simulink model "busrelay"  (Simulink 8.5)
settings: Solver=ode15s  SolverMode=SingleTasking  StartTime=0.0  StopTime=0.08  RelTol=1e-3  AbsTol=1e-6
libraries: powerlib_extras x27, elements x12
settings Model: Creator=PC  LastModifiedBy=PC  ExtModeTrigMode=oneshot  ExtModeArmWhenConnect=off
settings DataIOCC: LimitDataPoints=off
settings OptimizationCC: BlockReduction=off  BooleanDataType=off  ExpressionDepthLimit=128
settings DebuggingCC: SaveWithParameterizedLinksMsg=none  SignalResolutionControl=TryResolveAllWithWarning  MultiTaskDSMMsg=warning  MultiTaskCondExecSysMsg=none  FcnCallInpInsideContextMsg=EnableAllAsError  StateNameClashWarn=none  StrictBusMsg=None
settings HardwareCC: TargetUnknown=on

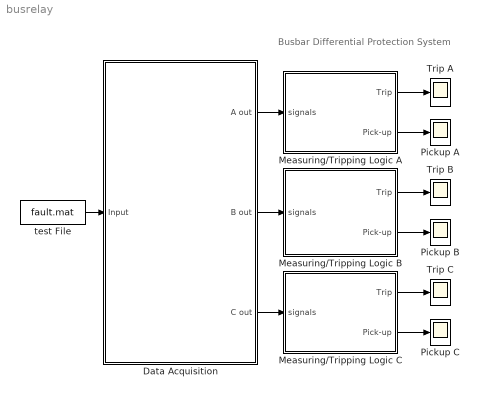
== system busrelay ==
  note: Busbar Differential Protection System
  Data Acquisition : Subsystem  mask(Data Acquisition Board){FreqSampling=60*20, FreqCutoff=360}
      mask prompts: FreqSampling "Sampling Frequecny (Hz) :"; FreqCutoff "Cut-off Frequency (Hz) :"
      mask Display: disp(' Data\nAcquistion\nBlock')
  Measuring/Tripping Logic A : Subsystem  mask(Biased Differential Relay){A0=0.2, Inorm=1, K=0.3, C1=0.1}
      mask prompts: A0 "Pickup Setting, A0 (pu):"; Inorm "Normal Load Current, Inorm (A) :"; K "Bias Setting, K (pu) :"; C1 "Harmonic Restrain Settging, C1 (pu)"
      mask help: coming soon ...
  Measuring/Tripping Logic B : Subsystem  mask(Biased Differential Relay){A0=0.2, Inorm=1, K=0.3, C1=0.1}
      mask prompts: A0 "Pickup Setting, A0 (pu):"; Inorm "Normal Load Current, Inorm (A) :"; K "Bias Setting, K (pu) :"; C1 "Harmonic Restrain Settging, C1 (pu)"
      mask help: coming soon ...
  Measuring/Tripping Logic C : Subsystem  mask(Biased Differential Relay){A0=0.2, Inorm=1, K=0.3, C1=0.1}
      mask prompts: A0 "Pickup Setting, A0 (pu):"; Inorm "Normal Load Current, Inorm (A) :"; K "Bias Setting, K (pu) :"; C1 "Harmonic Restrain Settging, C1 (pu)"
      mask help: coming soon ...
  Pickup A : Scope
      settings: TickLabels=on  YMin=0  YMax=2
  Pickup B : Scope
      settings: TickLabels=on  YMin=0  YMax=2
  Pickup C : Scope
      settings: TickLabels=on  YMin=0  YMax=2
  Trip A : Scope
      settings: TickLabels=on  YMin=0  YMax=2
  Trip B : Scope
      settings: TickLabels=on  YMin=0  YMax=1
  Trip C : Scope
      settings: TickLabels=on  YMin=0  YMax=1
  test File : FromFile  FileName=fault.mat  SampleTime=0
  wires:
  Measuring/Tripping Logic A/1(Trip) -> Trip A/1
  Measuring/Tripping Logic A/2(Pick-up) -> Pickup A/1
  test File/1 -> Data Acquisition/1("Input ")
  Data Acquisition/1(A out) -> Measuring/Tripping Logic A/1(signals)
  Measuring/Tripping Logic B/1(Trip) -> Trip B/1
  Measuring/Tripping Logic B/2(Pick-up) -> Pickup B/1
  Measuring/Tripping Logic C/1(Trip) -> Trip C/1
  Measuring/Tripping Logic C/2(Pick-up) -> Pickup C/1
  Data Acquisition/2(" B out") -> Measuring/Tripping Logic B/1(signals)
  Data Acquisition/3(C out) -> Measuring/Tripping Logic C/1(signals)

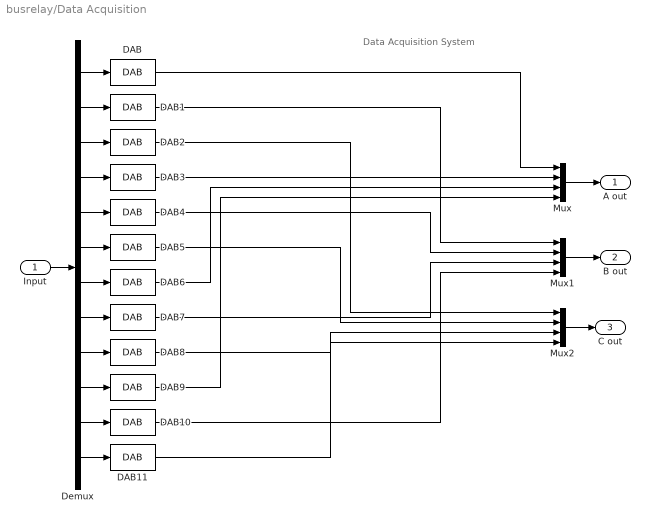
== system busrelay/Data Acquisition ==
  note: Data Acquisition System
  "Input " : Inport
  DAB{,1..11} (12 alike) : elements/DAB  filter=off  approx=Bessel  order=2  numerator=[]  denominator=[]  freq=FreqCutoff  resdis=off  vertres=12  xmax=10  winsize=1  G=1.0  fs=FreqSampling
  Demux : Demux  Outputs=12
  Mux : Mux
  Mux1 : Mux
  Mux2 : Mux
  A out : Outport
  " B out" : Outport  Port=2
  C out : Outport  Port=3
  wires:
  "Input "/1 -> Demux/1
  Mux/1 -> A out/1
  Mux2/1 -> C out/1
  Mux1/1 -> " B out"/1
  Demux/1 -> DAB/1
  DAB/1 -> Mux/1
  Demux/2 -> DAB1/1
  DAB1/1 -> Mux1/1
  Demux/3 -> DAB2/1
  DAB2/1 -> Mux2/1
  Demux/4 -> DAB3/1
  DAB3/1 -> Mux/2
  Demux/5 -> DAB4/1
  DAB4/1 -> Mux1/2
  Demux/6 -> DAB5/1
  DAB5/1 -> Mux2/2
  Demux/7 -> DAB6/1
  DAB6/1 -> Mux/3
  Demux/8 -> DAB7/1
  DAB7/1 -> Mux1/3
  Demux/9 -> DAB8/1
  Demux/10 -> DAB9/1
  DAB9/1 -> Mux/4
  Demux/11 -> DAB10/1
  DAB10/1 -> Mux1/4
  Demux/12 -> DAB11/1
  DAB11/1 -> Mux2/4
  DAB8/1 -> Mux2/3

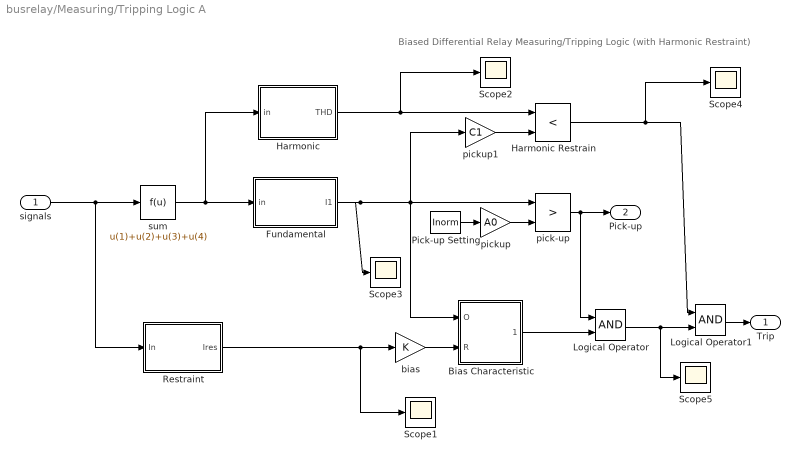
== system busrelay/Measuring/Tripping Logic A ==
  note: Biased Differential Relay Measuring/Tripping Logic (with Harmonic Restraint)
  signals : Inport
  Bias Characteristic : Subsystem  mask(Bias Characteristic){BC=[0 0;0 0.3; 0.1 0.8 ;7 4.2], fs=60*20}
      mask prompts: BC "Bias characteristic"; fs "Sampling frequency [samples per cycle]"
      mask help: Compares its two input signals using a bias characteristic. This characteristic is defined point-by-point.
      mask init:
      | bc2
      mask Display:
      | plot([xo xo],[yo y1]);
      | plot([xo x1],[yo yo]);
      | 
      | 
      | plot(R,O);
  Fundamental : Subsystem
  Harmonic : Subsystem
  Harmonic Restrain : RelationalOperator  Operator=<  InputSameDT=on
  Logical Operator : Logic
  Logical Operator1 : Logic
  Pick-up Setting : Constant  Value=Inorm
  Restraint : Subsystem
  Scope{1..5} (5 alike) : Scope
      settings: TickLabels=on  YMin=0  YMax=1
  bias : Gain  Gain=K  SaturateOnIntegerOverflow=on  OutDataTypeStr=Inherit: Same as input  ParamDataTypeStr=Inherit: Same as input
  pick-up : RelationalOperator  Operator=>  InputSameDT=on
  pickup : Gain  Gain=A0  SaturateOnIntegerOverflow=on  OutDataTypeStr=Inherit: Same as input  ParamDataTypeStr=Inherit: Same as input
  pickup1 : Gain  Gain=C1  SaturateOnIntegerOverflow=on  OutDataTypeStr=Inherit: Same as input  ParamDataTypeStr=Inherit: Same as input
  sum : Fcn  Expr=u(1)+u(2)+u(3)+u(4)
  Trip : Outport
  Pick-up : Outport  Port=2
  wires:
  signals/1 -> sum/1, Restraint/1(In)
  bias/1 -> Bias Characteristic/2(R)
  Restraint/1(Ires) -> bias/1, Scope1/1
  Bias Characteristic/1(" ") -> Logical Operator/2
  sum/1 -> Harmonic/1(in), Fundamental/1(in)
  pickup1/1 -> Harmonic Restrain/2
  Logical Operator1/1 -> Trip/1
  Pick-up Setting/1 -> pickup/1
  pickup/1 -> pick-up/2
  pick-up/1 -> Pick-up/1, Logical Operator/1
  Harmonic/1(THD) -> Harmonic Restrain/1, Scope2/1
  Fundamental/1(I1) -> pick-up/1, Bias Characteristic/1(O), pickup1/1, Scope3/1
  Harmonic Restrain/1 -> Logical Operator1/1, Scope4/1
  Logical Operator/1 -> Logical Operator1/2, Scope5/1

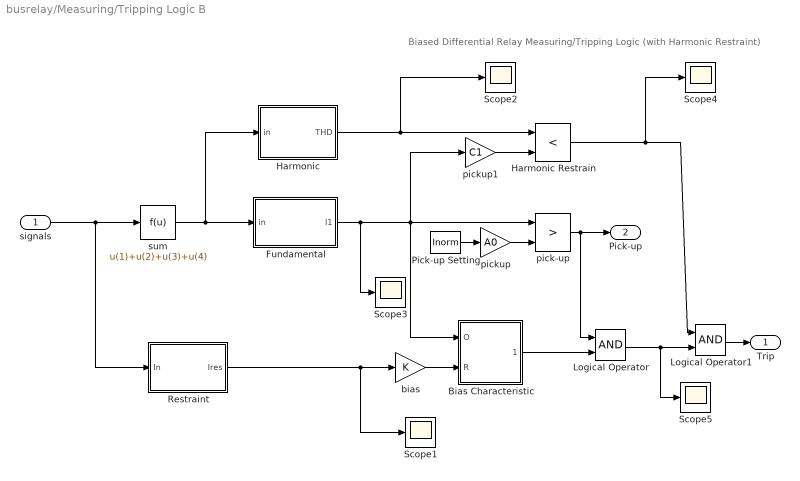
== system busrelay/Measuring/Tripping Logic B ==
  note: Biased Differential Relay Measuring/Tripping Logic (with Harmonic Restraint)
  signals : Inport
  Bias Characteristic : Subsystem  mask(Bias Characteristic){BC=[0 0;0 0.3; 0.1 0.8 ;7 4.2], fs=60*20}
      mask prompts: BC "Bias characteristic"; fs "Sampling frequency [samples per cycle]"
      mask help: Compares its two input signals using a bias characteristic. This characteristic is defined point-by-point.
      mask init:
      | bc2
      mask Display:
      | plot([xo xo],[yo y1]);
      | plot([xo x1],[yo yo]);
      | 
      | 
      | plot(R,O);
  Fundamental : Subsystem
  Harmonic : Subsystem
  Harmonic Restrain : RelationalOperator  Operator=<  InputSameDT=on
  Logical Operator : Logic
  Logical Operator1 : Logic
  Pick-up Setting : Constant  Value=Inorm
  Restraint : Subsystem
  Scope{1..5} (5 alike) : Scope
      settings: TickLabels=on  YMin=0  YMax=1
  bias : Gain  Gain=K  SaturateOnIntegerOverflow=on  OutDataTypeStr=Inherit: Same as input  ParamDataTypeStr=Inherit: Same as input
  pick-up : RelationalOperator  Operator=>  InputSameDT=on
  pickup : Gain  Gain=A0  SaturateOnIntegerOverflow=on  OutDataTypeStr=Inherit: Same as input  ParamDataTypeStr=Inherit: Same as input
  pickup1 : Gain  Gain=C1  SaturateOnIntegerOverflow=on  OutDataTypeStr=Inherit: Same as input  ParamDataTypeStr=Inherit: Same as input
  sum : Fcn  Expr=u(1)+u(2)+u(3)+u(4)
  Trip : Outport
  Pick-up : Outport  Port=2
  wires:
  Logical Operator/1 -> Scope5/1, Logical Operator1/2
  Harmonic Restrain/1 -> Scope4/1, Logical Operator1/1
  Fundamental/1(I1) -> Scope3/1, pickup1/1, Bias Characteristic/1(O), pick-up/1
  Harmonic/1(THD) -> Scope2/1, Harmonic Restrain/1
  pick-up/1 -> Logical Operator/1, Pick-up/1
  pickup/1 -> pick-up/2
  Pick-up Setting/1 -> pickup/1
  Logical Operator1/1 -> Trip/1
  pickup1/1 -> Harmonic Restrain/2
  sum/1 -> Fundamental/1(in), Harmonic/1(in)
  Bias Characteristic/1(" ") -> Logical Operator/2
  Restraint/1(Ires) -> Scope1/1, bias/1
  bias/1 -> Bias Characteristic/2(R)
  signals/1 -> Restraint/1(In), sum/1

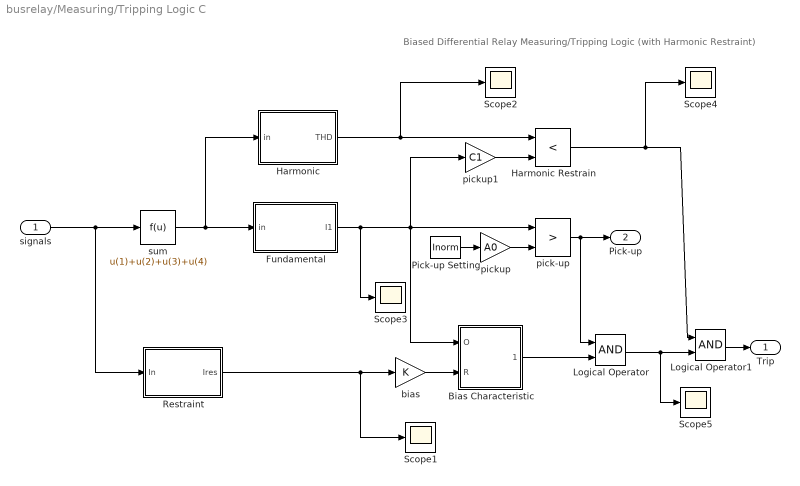
== system busrelay/Measuring/Tripping Logic C ==
  note: Biased Differential Relay Measuring/Tripping Logic (with Harmonic Restraint)
  signals : Inport
  Bias Characteristic : Subsystem  mask(Bias Characteristic){BC=[0 0;0 0.3; 0.1 0.8 ;7 4.2], fs=60*20}
      mask prompts: BC "Bias characteristic"; fs "Sampling frequency [samples per cycle]"
      mask help: Compares its two input signals using a bias characteristic. This characteristic is defined point-by-point.
      mask init:
      | bc2
      mask Display:
      | plot([xo xo],[yo y1]);
      | plot([xo x1],[yo yo]);
      | 
      | 
      | plot(R,O);
  Fundamental : Subsystem
  Harmonic : Subsystem
  Harmonic Restrain : RelationalOperator  Operator=<  InputSameDT=on
  Logical Operator : Logic
  Logical Operator1 : Logic
  Pick-up Setting : Constant  Value=Inorm
  Restraint : Subsystem
  Scope{1..5} (5 alike) : Scope
      settings: TickLabels=on  YMin=0  YMax=1
  bias : Gain  Gain=K  SaturateOnIntegerOverflow=on  OutDataTypeStr=Inherit: Same as input  ParamDataTypeStr=Inherit: Same as input
  pick-up : RelationalOperator  Operator=>  InputSameDT=on
  pickup : Gain  Gain=A0  SaturateOnIntegerOverflow=on  OutDataTypeStr=Inherit: Same as input  ParamDataTypeStr=Inherit: Same as input
  pickup1 : Gain  Gain=C1  SaturateOnIntegerOverflow=on  OutDataTypeStr=Inherit: Same as input  ParamDataTypeStr=Inherit: Same as input
  sum : Fcn  Expr=u(1)+u(2)+u(3)+u(4)
  Trip : Outport
  Pick-up : Outport  Port=2
  wires:
  signals/1 -> sum/1, Restraint/1(In)
  bias/1 -> Bias Characteristic/2(R)
  Restraint/1(Ires) -> bias/1, Scope1/1
  Bias Characteristic/1(" ") -> Logical Operator/2
  sum/1 -> Harmonic/1(in), Fundamental/1(in)
  pickup1/1 -> Harmonic Restrain/2
  Logical Operator1/1 -> Trip/1
  Pick-up Setting/1 -> pickup/1
  pickup/1 -> pick-up/2
  pick-up/1 -> Pick-up/1, Logical Operator/1
  Harmonic/1(THD) -> Harmonic Restrain/1, Scope2/1
  Fundamental/1(I1) -> pick-up/1, Bias Characteristic/1(O), pickup1/1, Scope3/1
  Harmonic Restrain/1 -> Logical Operator1/1, Scope4/1
  Logical Operator/1 -> Logical Operator1/2, Scope5/1

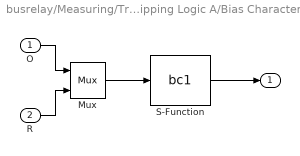
== system busrelay/Measuring/Tripping Logic A/Bias Characteristic ==
  O : Inport
  R : Inport  Port=2
  Mux : Mux  Inputs=2
  S-Function : S-Function  FunctionName=bc1  Parameters=BC,fs
  " " : Outport
  wires:
  S-Function/1 -> " "/1
  O/1 -> Mux/1
  R/1 -> Mux/2
  Mux/1 -> S-Function/1

== system busrelay/Measuring/Tripping Logic A/Fundamental ==
  in : Inport
  Fourier : powerlib_extras/Measurements/Fourier  f1=60  n=1
  Terminator : Terminator
  I1 : Outport
  wires:
  Fourier/2 -> Terminator/1
  in/1 -> Fourier/1
  Fourier/1 -> I1/1

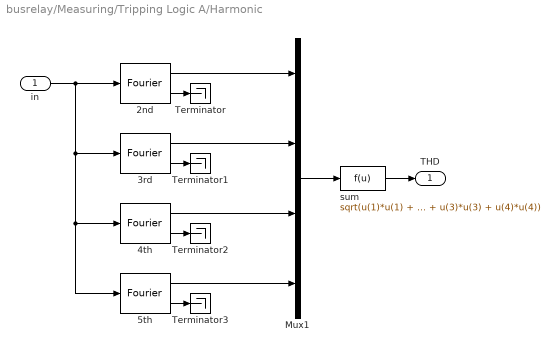
== system busrelay/Measuring/Tripping Logic A/Harmonic ==
  in : Inport
  2nd : powerlib_extras/Measurements/Fourier  f1=60  n=2
  3rd : powerlib_extras/Measurements/Fourier  f1=60  n=3
  4th : powerlib_extras/Measurements/Fourier  f1=60  n=4
  5th : powerlib_extras/Measurements/Fourier  f1=60  n=5
  Mux1 : Mux
  Terminator{,1..3} (4 alike) : Terminator
  sum : Fcn  Expr=sqrt(u(1)*u(1) + u(2)*u(2) + u(3)*u(3) + u(4)*u(4))
  THD : Outport
  wires:
  in/1 -> 2nd/1, 3rd/1, 5th/1, 4th/1
  2nd/2 -> Terminator/1
  2nd/1 -> Mux1/1
  3rd/2 -> Terminator1/1
  3rd/1 -> Mux1/2
  4th/2 -> Terminator2/1
  4th/1 -> Mux1/3
  5th/2 -> Terminator3/1
  5th/1 -> Mux1/4
  Mux1/1 -> sum/1
  sum/1 -> THD/1

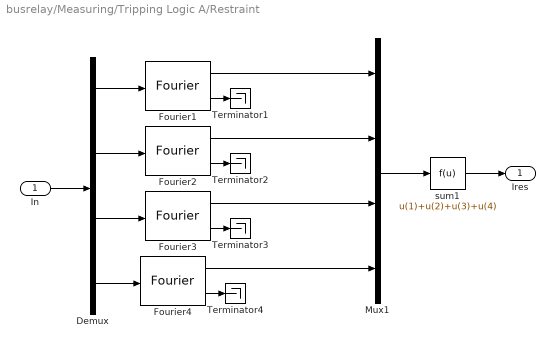
== system busrelay/Measuring/Tripping Logic A/Restraint ==
  In : Inport
  Demux : Demux
  Fourier{1..4} (4 alike) : powerlib_extras/Measurements/Fourier  f1=60  n=1
  Mux1 : Mux
  Terminator{1..4} (4 alike) : Terminator
  sum1 : Fcn  Expr=u(1)+u(2)+u(3)+u(4)
  Ires : Outport
  wires:
  Demux/1 -> Fourier1/1
  Fourier1/2 -> Terminator1/1
  Fourier1/1 -> Mux1/1
  In/1 -> Demux/1
  Fourier2/2 -> Terminator2/1
  Fourier2/1 -> Mux1/2
  Demux/2 -> Fourier2/1
  Fourier3/2 -> Terminator3/1
  Fourier3/1 -> Mux1/3
  Demux/3 -> Fourier3/1
  Fourier4/2 -> Terminator4/1
  Fourier4/1 -> Mux1/4
  Demux/4 -> Fourier4/1
  Mux1/1 -> sum1/1
  sum1/1 -> Ires/1

== system busrelay/Measuring/Tripping Logic B/Bias Characteristic ==
  O : Inport
  R : Inport  Port=2
  Mux : Mux  Inputs=2
  S-Function : S-Function  FunctionName=bc1  Parameters=BC,fs
  " " : Outport
  wires:
  Mux/1 -> S-Function/1
  R/1 -> Mux/2
  O/1 -> Mux/1
  S-Function/1 -> " "/1

== system busrelay/Measuring/Tripping Logic B/Fundamental ==
  in : Inport
  Fourier : powerlib_extras/Measurements/Fourier  f1=60  n=1
  Terminator : Terminator
  I1 : Outport
  wires:
  Fourier/1 -> I1/1
  in/1 -> Fourier/1
  Fourier/2 -> Terminator/1

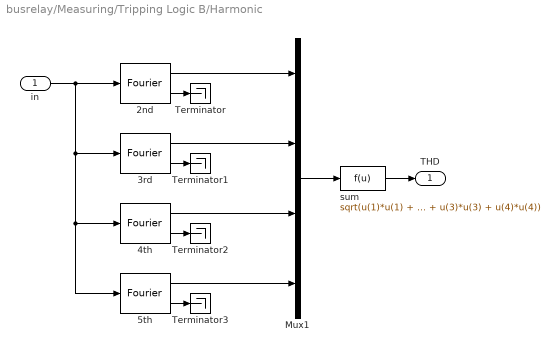
== system busrelay/Measuring/Tripping Logic B/Harmonic ==
  in : Inport
  2nd : powerlib_extras/Measurements/Fourier  f1=60  n=2
  3rd : powerlib_extras/Measurements/Fourier  f1=60  n=3
  4th : powerlib_extras/Measurements/Fourier  f1=60  n=4
  5th : powerlib_extras/Measurements/Fourier  f1=60  n=5
  Mux1 : Mux
  Terminator{,1..3} (4 alike) : Terminator
  sum : Fcn  Expr=sqrt(u(1)*u(1) + u(2)*u(2) + u(3)*u(3) + u(4)*u(4))
  THD : Outport
  wires:
  sum/1 -> THD/1
  Mux1/1 -> sum/1
  5th/1 -> Mux1/4
  5th/2 -> Terminator3/1
  4th/1 -> Mux1/3
  4th/2 -> Terminator2/1
  3rd/1 -> Mux1/2
  3rd/2 -> Terminator1/1
  2nd/1 -> Mux1/1
  2nd/2 -> Terminator/1
  in/1 -> 4th/1, 5th/1, 3rd/1, 2nd/1

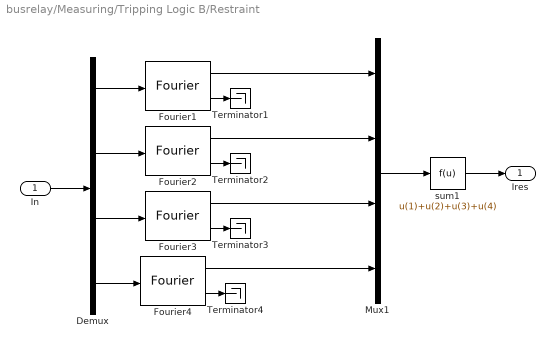
== system busrelay/Measuring/Tripping Logic B/Restraint ==
  In : Inport
  Demux : Demux
  Fourier{1..4} (4 alike) : powerlib_extras/Measurements/Fourier  f1=60  n=1
  Mux1 : Mux
  Terminator{1..4} (4 alike) : Terminator
  sum1 : Fcn  Expr=u(1)+u(2)+u(3)+u(4)
  Ires : Outport
  wires:
  sum1/1 -> Ires/1
  Mux1/1 -> sum1/1
  Demux/4 -> Fourier4/1
  Fourier4/1 -> Mux1/4
  Fourier4/2 -> Terminator4/1
  Demux/3 -> Fourier3/1
  Fourier3/1 -> Mux1/3
  Fourier3/2 -> Terminator3/1
  Demux/2 -> Fourier2/1
  Fourier2/1 -> Mux1/2
  Fourier2/2 -> Terminator2/1
  In/1 -> Demux/1
  Fourier1/1 -> Mux1/1
  Fourier1/2 -> Terminator1/1
  Demux/1 -> Fourier1/1

== system busrelay/Measuring/Tripping Logic C/Bias Characteristic ==
  O : Inport
  R : Inport  Port=2
  Mux : Mux  Inputs=2
  S-Function : S-Function  FunctionName=bc1  Parameters=BC,fs
  " " : Outport
  wires:
  S-Function/1 -> " "/1
  O/1 -> Mux/1
  R/1 -> Mux/2
  Mux/1 -> S-Function/1

== system busrelay/Measuring/Tripping Logic C/Fundamental ==
  in : Inport
  Fourier : powerlib_extras/Measurements/Fourier  f1=60  n=1
  Terminator : Terminator
  I1 : Outport
  wires:
  Fourier/2 -> Terminator/1
  in/1 -> Fourier/1
  Fourier/1 -> I1/1

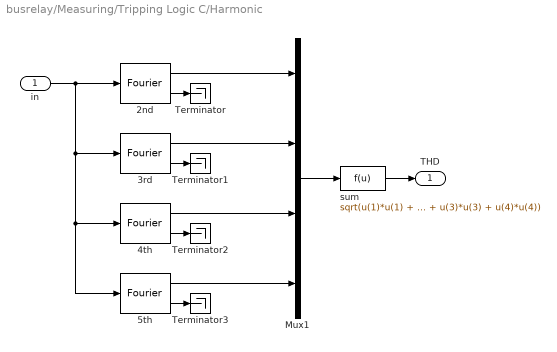
== system busrelay/Measuring/Tripping Logic C/Harmonic ==
  in : Inport
  2nd : powerlib_extras/Measurements/Fourier  f1=60  n=2
  3rd : powerlib_extras/Measurements/Fourier  f1=60  n=3
  4th : powerlib_extras/Measurements/Fourier  f1=60  n=4
  5th : powerlib_extras/Measurements/Fourier  f1=60  n=5
  Mux1 : Mux
  Terminator{,1..3} (4 alike) : Terminator
  sum : Fcn  Expr=sqrt(u(1)*u(1) + u(2)*u(2) + u(3)*u(3) + u(4)*u(4))
  THD : Outport
  wires:
  in/1 -> 2nd/1, 3rd/1, 5th/1, 4th/1
  2nd/2 -> Terminator/1
  2nd/1 -> Mux1/1
  3rd/2 -> Terminator1/1
  3rd/1 -> Mux1/2
  4th/2 -> Terminator2/1
  4th/1 -> Mux1/3
  5th/2 -> Terminator3/1
  5th/1 -> Mux1/4
  Mux1/1 -> sum/1
  sum/1 -> THD/1

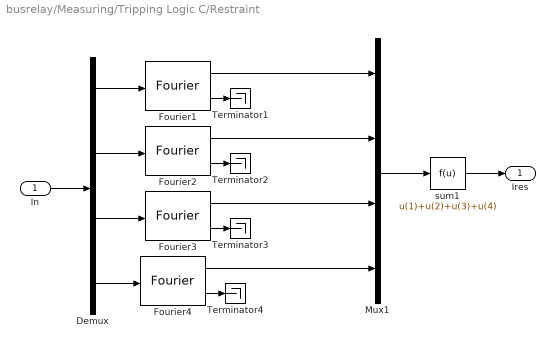
== system busrelay/Measuring/Tripping Logic C/Restraint ==
  In : Inport
  Demux : Demux
  Fourier{1..4} (4 alike) : powerlib_extras/Measurements/Fourier  f1=60  n=1
  Mux1 : Mux
  Terminator{1..4} (4 alike) : Terminator
  sum1 : Fcn  Expr=u(1)+u(2)+u(3)+u(4)
  Ires : Outport
  wires:
  Demux/1 -> Fourier1/1
  Fourier1/2 -> Terminator1/1
  Fourier1/1 -> Mux1/1
  In/1 -> Demux/1
  Fourier2/2 -> Terminator2/1
  Fourier2/1 -> Mux1/2
  Demux/2 -> Fourier2/1
  Fourier3/2 -> Terminator3/1
  Fourier3/1 -> Mux1/3
  Demux/3 -> Fourier3/1
  Fourier4/2 -> Terminator4/1
  Fourier4/1 -> Mux1/4
  Demux/4 -> Fourier4/1
  Mux1/1 -> sum1/1
  sum1/1 -> Ires/1
